simulink model "sistema_fuzzy"  (Simulink 7.5)
settings: Solver=ode45  StartTime=0.0  StopTime=100.0  RelTol=1e-3
libraries: fuzblock x1
settings Model: Creator=manu  LastModifiedBy=manu

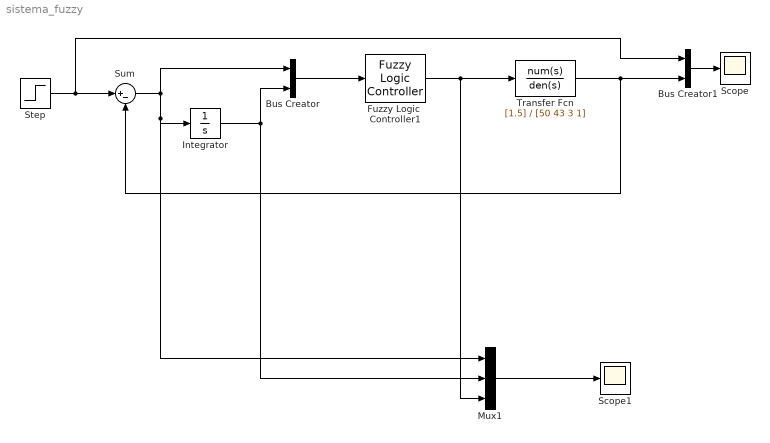
== system sistema_fuzzy ==
  Bus Creator : BusCreator  Inputs=2
  Bus Creator1 : BusCreator  Inputs=2
  Fuzzy Logic  Controller1 : fuzblock/Fuzzy Logic  Controller  SystemSampleTime=-1  fis='sistema_mamdani.fis'
  Integrator : Integrator
  Mux1 : Mux  Inputs=3
  Scope : Scope
      settings: YMin=-0.5  YMax=1.1
  Scope1 : Scope
      settings: TimeRange=100  YMin=0  YMax=1.4
  Step : Step  SampleTime=0
  Sum : Sum  Inputs=|+-
  Transfer Fcn : TransferFcn  Numerator=[1.5]  Denominator=[50 43 3 1]
  wires:
  Fuzzy Logic  Controller1/1 -> Transfer Fcn/1, Mux1/3
  Sum/1 -> Bus Creator/1, Integrator/1, Mux1/1
  Bus Creator/1 -> Fuzzy Logic  Controller1/1
  Transfer Fcn/1 -> Sum/2, Bus Creator1/2
  Step/1 -> Sum/1, Bus Creator1/1
  Bus Creator1/1 -> Scope/1
  Integrator/1 -> Bus Creator/2, Mux1/2
  Mux1/1 -> Scope1/1
